simulink model "nncACCsystem_5_50"  (R2021a)
(part 13 of 14)

  "IW{5,4}(50,:)'" : Constant  Value=[0.1141432004020616342021554601160460151731967926025390625;-0.017584047457666528158082286381613812409341335296630859375;0.66805155463235965651591641289996914565563201904296875;-0.6136001546513243365410517071723006665706634521484375;0.95937034133340282071600313429371453821659088134765625;0.075971577456444838727378510156995616853237152099609375;0.5297921278961776891947010881267488002777099609375;0.12067691519441682557189920999007881619036197662353515625;-0.191581829978980433537572025670669972896575927734375;-0.1087005623838290524485472587912227027118206024169921875;0.0784168938973104356904286760254763066768646240234375;0.6065395454377213724228568025864660739898681640625;-0.346902780311276026647959724868997000157833099365234375;0.217804850814769912492607772946939803659915924072265625;-0.990997053395485050231172863277606666088104248046875;0.0857487248848738670137237249946338124573230743408203125;-0.05128831403013651979438947137168725021183490753173828125;-0.9629031136673800173042536698631010949611663818359375;-0.829893972023025838780085905455052852630615234375;-0.74057440662256468488777727543492801487445831298828125;0.5856000846022102468424463950213976204395294189453125;0.515406069917983433725794384372420608997344970703125;0.8084890601401026888339629294932819902896881103515625;0.21723000990280361133244468874181620776653289794921875;-0.211007213040456775843267678283154964447021484375;-0.52450505825967430606482366783893667161464691162109375;-0.7760978893070304973633710687863640487194061279296875;-0.2729152713620124348636863942374475300312042236328125;-0.7843894258724890544698382655042223632335662841796875;0.7267607104040860743765506413183175027370452880859375;0.06688400233054224430784273636163561604917049407958984375;-0.22242900136235022046093945391476154327392578125;-0.433234064722516354351000700262375175952911376953125;0.268465430229838819542464989353902637958526611328125;0.83968421280373828352594500756822526454925537109375;-0.300231039082238027049243100918829441070556640625;-0.50942280050992094775352825308800674974918365478515625;-0.072633643631129007900426586274988949298858642578125;-0.0176651529053561962001595020410604774951934814453125;-0.1689808965722979505752476825364283286035060882568359375;-0.61101340370974821514238328745705075562000274658203125;-0.92770092769464718163163752251421101391315460205078125;-0.6814966471176699958078870622557587921619415283203125;0.74963349363538289704678163616335950791835784912109375;0.471918139959748739187261890037916600704193115234375;0.42976609261675891016096784369437955319881439208984375;-0.2913539067186416975374640969675965607166290283203125;-0.26473179229769050468945579268620349466800689697265625;-0.1494398826271263747145212619216181337833404541015625;-0.0047963111412494228991132416695108986459672451019287109375]
      mask Display: e = 0.06;c1 = [120 150 230]/255;c2 = ([120 150 230]+0)/383;c3 = ([120 150 230]+128)/383;patch([0 1 1 0],[0 0 1 1],c1);patch([0 1 1 1-e 1-e 0+e],[0 0 1 1-e 0+e 0+e],c2);patch([0 0 1 1-e 0+e 0+e],[0 1 1 1-e 1-e 0+e],c3);plot([0 1 1 0 0],[0 0 1 1 0]);disp('weights');
  "IW{5,4}(6,:)'" : Constant  Value=[0.3562295317008794537372295962995849549770355224609375;-0.9594267744298006217462670974782668054103851318359375;-0.8561211729585240792772538043209351599216461181640625;-0.6858649005114350050149596427218057215213775634765625;0.693357420721138151264995030942372977733612060546875;0.6491811538530491976217717819963581860065460205078125;0.4650031948144783822129966210923157632350921630859375;-0.4006238615764019517229144184966571629047393798828125;-0.8360217807908802978289486418361775577068328857421875;-0.0467611414599111707701695195282809436321258544921875;-0.901853552230166055636573219089768826961517333984375;-0.350978204962510975661871270858682692050933837890625;-0.2877242832576334397032269407645799219608306884765625;0.0514980364986763472501252181245945394039154052734375;0.26081748415533212437367183156311511993408203125;0.3529120801958651743035488834721036255359649658203125;0.6029519225999704357121800057939253747463226318359375;-0.0818034610827227393059501991956494748592376708984375;0.134101733301195569225683357217349112033843994140625;-0.6303215523613399096092280160519294440746307373046875;-0.79676277486145608008882845751941204071044921875;0.4374804970924806024612507826532237231731414794921875;0.1479652196327256863384036478237248957157135009765625;0.0855815758666143011623717029578983783721923828125;-0.8378126628961728439293210612959228456020355224609375;-0.6633050510598119675620409907423891127109527587890625;-0.8438418931206477235917873258586041629314422607421875;-0.828178424658374989775211361120454967021942138671875;0.7593314799986021768063437775708734989166259765625;0.1850531885661881315030541372834704816341400146484375;0.01103491414841784035161253996193408966064453125;0.0433833817025632839659010642208158969879150390625;-0.3893360678296999832781466466258279979228973388671875;0.1383580395647197036623765598051249980926513671875;-0.2893368068265278481021596235223114490509033203125;0.6991119862498920145554848204483278095722198486328125;-0.8131628013724869763478864115313626825809478759765625;0.786580773429571333821286316378973424434661865234375;0.0515801109804245871970351799973286688327789306640625;-0.2752704126105511850397533635259605944156646728515625;-0.0373661458551948211237458963296376168727874755859375;0.4458566657836804392189833379234187304973602294921875;-0.656736574649199322806225609383545815944671630859375;0.2401126867635745565365823495085351169109344482421875;-0.8042628758426690893656996195204555988311767578125;-0.95927744782383772559342105523683130741119384765625;-0.82736867483109488574655188131146132946014404296875;-0.66927779776266316247301801922731101512908935546875;-0.0234373844901714090127597955870442092418670654296875;-0.0099647596443699359980428198468871414661407470703125]
      mask Display: e = 0.06;c1 = [120 150 230]/255;c2 = ([120 150 230]+0)/383;c3 = ([120 150 230]+128)/383;patch([0 1 1 0],[0 0 1 1],c1);patch([0 1 1 1-e 1-e 0+e],[0 0 1 1-e 0+e 0+e],c2);patch([0 0 1 1-e 0+e 0+e],[0 1 1 1-e 1-e 0+e],c3);plot([0 1 1 0 0],[0 0 1 1 0]);disp('weights');
  "IW{5,4}(7,:)'" : Constant  Value=[-0.501231035064013230595492132124491035938262939453125;-0.357691629081013429125590619150898419320583343505859375;-0.7900913539664988771704656755900941789150238037109375;0.2096838828164602208659061943762935698032379150390625;0.62382138299157607885803145109093748033046722412109375;0.1366901035758718296886371490472811274230480194091796875;-0.233367237568067320552245291764847934246063232421875;0.252547828187033640556791169728967361152172088623046875;0.7087636839718935988230441580526530742645263671875;-0.90527397696553568717803273102617822587490081787109375;0.6014760521333943898980578524060547351837158203125;-0.530859910497331721757063860422931611537933349609375;-0.38246638282558509391861889525898732244968414306640625;0.31591269256083831518111537661752663552761077880859375;-0.62210156570651020668805131208500824868679046630859375;-0.480663856403305889131161166005767881870269775390625;0.0945553776214251018306100604604580439627170562744140625;-0.1882986261857273191377970533721963874995708465576171875;0.152877254705158893699490363360382616519927978515625;-0.0699828261606157686625095948329544626176357269287109375;-0.58808697276489441119196044382988475263118743896484375;0.357367299668190085970564950912375934422016143798828125;0.70759581042943209272522153696627356112003326416015625;-0.042104488211461947588798437891455250792205333709716796875;-0.5940109083731683892182218187372200191020965576171875;0.85650981721000807311838798341341316699981689453125;0.3521252772321890045503778310376219451427459716796875;0.81358484949936660246549990915809758007526397705078125;-0.718740687327045879584375143167562782764434814453125;-0.331609948990100489307764064506045542657375335693359375;0.5977500263709998318262250904808752238750457763671875;-0.375894633733153238352997504989616572856903076171875;-0.80113567733840085338670178316533565521240234375;0.7216532547682579235015509766526520252227783203125;0.8335636424205983274760001222603023052215576171875;-0.4197666285151575582546001896844245493412017822265625;0.63216733030109562019305258218082599341869354248046875;-0.1751530510027360654223826941233710385859012603759765625;0.5914122117394067235096599688404239714145660400390625;0.1766025750526220294833734669737168587744235992431640625;0.353507921430033345000509825695189647376537322998046875;-0.884736247267077668965384873445145785808563232421875;0.0273307323542046898268154109246097505092620849609375;0.16360477382383231681473034768714569509029388427734375;-0.854591073876117324203960379236377775669097900390625;-0.55889232599558991143595676476252265274524688720703125;-0.850124795777536856888900729245506227016448974609375;0.9188706920610811845762100347201339900493621826171875;-0.0448718826156000449856264822301454842090606689453125;-0.071636817070096336923512581051909364759922027587890625]
      mask Display: e = 0.06;c1 = [120 150 230]/255;c2 = ([120 150 230]+0)/383;c3 = ([120 150 230]+128)/383;patch([0 1 1 0],[0 0 1 1],c1);patch([0 1 1 1-e 1-e 0+e],[0 0 1 1-e 0+e 0+e],c2);patch([0 0 1 1-e 0+e 0+e],[0 1 1 1-e 1-e 0+e],c3);plot([0 1 1 0 0],[0 0 1 1 0]);disp('weights');
  "IW{5,4}(8,:)'" : Constant  Value=[-0.835397376692058823977049542008899152278900146484375;-0.1863177926218158031446137101738713681697845458984375;0.947840470946463842238927099970169365406036376953125;-0.40320951499648050031510138069279491901397705078125;0.8429824173771149897760324165574274957180023193359375;0.189470039698699910246659783297218382358551025390625;-0.168120473083930743740666002850048243999481201171875;0.3850826533089504177809203611104749143123626708984375;-0.0568519217815877109245548126637004315853118896484375;0.8730703813938365254188056496786884963512420654296875;-0.76807973930514084059950619121082127094268798828125;0.985893388329737607733704862766899168491363525390625;0.957910694214652469469228890375234186649322509765625;0.567445330118751645187558096949942409992218017578125;-0.073250503132566091579747080686502158641815185546875;-0.2572748304222669535334944157511927187442779541015625;-0.9233194436739300403615970935788936913013458251953125;0.693241279306989088837553936173208057880401611328125;-0.7155330006054583247276923430035822093486785888671875;-0.6614285298641149335452382729272358119487762451171875;-0.1588593543599252644327179950778372585773468017578125;0.2010344578168161699949223475414328277111053466796875;-0.1237958922126274341479756913031451404094696044921875;-0.1151649177598332851601981019484810531139373779296875;-0.49354322715469667315346669056452810764312744140625;-0.702844637054997445346771201002411544322967529296875;0.65052194756236314532316100667230784893035888671875;-0.333695281534292842451350225019268691539764404296875;0.761133946108828229881737570394761860370635986328125;-0.1631563584736659411333903335616923868656158447265625;-0.75700179216406393578608913230709731578826904296875;-0.449358337881843095118483688565902411937713623046875;-0.790585520472188107987676630727946758270263671875;-0.5439977754440203927543961981427855789661407470703125;-0.4510031405965089223997210865491069853305816650390625;-0.4421511393272237189222551023703999817371368408203125;-0.025489463464555495164631793159060180187225341796875;-0.3536782445976800470788248276221565902233123779296875;-0.307989351103557407185462579946033656597137451171875;-0.5623830419630575505607339437119662761688232421875;0.58988972588036858724080957472324371337890625;-0.4032539307774827275210327570675872266292572021484375;0.4908366314473247005167877432540990412235260009765625;0.003280045227161298981854997691698372364044189453125;-0.3422400378460412895265108090825378894805908203125;-0.721939022319336487498731003142893314361572265625;-0.1268024164893539751375328705762512981891632080078125;-0.5045654316656384974493221307056955993175506591796875;-0.9188881947066196431705975555814802646636962890625;0.2464410919689814516431169977295212447643280029296875]
      mask Display: e = 0.06;c1 = [120 150 230]/255;c2 = ([120 150 230]+0)/383;c3 = ([120 150 230]+128)/383;patch([0 1 1 0],[0 0 1 1],c1);patch([0 1 1 1-e 1-e 0+e],[0 0 1 1-e 0+e 0+e],c2);patch([0 0 1 1-e 0+e 0+e],[0 1 1 1-e 1-e 0+e],c3);plot([0 1 1 0 0],[0 0 1 1 0]);disp('weights');
  "IW{5,4}(9,:)'" : Constant  Value=[0.125263869427104879150647320784628391265869140625;-0.26892420971510777594204455454018898308277130126953125;-0.336354899111460048377608700320706702768802642822265625;-0.904315649536205246050712958094663918018341064453125;-0.88276543462096912495695733014144934713840484619140625;0.1946548813334317562517838950952864252030849456787109375;-0.507868156492297107007516387966461479663848876953125;0.9092107987620712261644939644611440598964691162109375;0.721076330649817354156994042568840086460113525390625;0.6995281039499550157501062130904756486415863037109375;0.768981913009282092019702758989296853542327880859375;0.8510055912506089281777121868799440562725067138671875;0.9110055475525749013598897363408468663692474365234375;-0.1512888880825329074308882582045043818652629852294921875;0.9864111784332727506097171499277465045452117919921875;0.45705781453436333805484537151642143726348876953125;0.0582522255673158240174558386570424772799015045166015625;-0.2783090350975634397201474712346680462360382080078125;-0.2050213130668951944102218476473353803157806396484375;0.9062783858765453004480150411836802959442138671875;-0.2275372272443366428174016391494660638272762298583984375;-0.74975055782701927054034740649512968957424163818359375;-0.00167456629070278297140295098444084942457266151905059814453125;-0.68684648197941322589343826621188782155513763427734375;0.274321371547895154208163148723542690277099609375;-0.8326166588818690872386696355533786118030548095703125;0.3492783513319797084051288038608618080615997314453125;-0.352424262757165263071357230728608556091785430908203125;-0.56161177963944464153200897271744906902313232421875;0.60711015775531829152811269523226656019687652587890625;0.653327372178704735006249393336474895477294921875;-0.2734280753837075028656045105890370905399322509765625;0.9471567103199796111567820844356901943683624267578125;0.0691495345151629248192648447002284228801727294921875;-0.55269637080893829761407687328755855560302734375;0.8364099330009135968566624796949326992034912109375;0.93565814778570077780983638149336911737918853759765625;0.7440300375040942437721014357521198689937591552734375;-0.6031580020371298811454607857740484178066253662109375;0.54771961519984102562119687718222849071025848388671875;0.356311952272694298926580813713371753692626953125;-0.23858451746665476633779690018855035305023193359375;0.369998883276509094031325730611570179462432861328125;-0.9154668776852885603290133076370693743228912353515625;0.32110909552635202857118201791308820247650146484375;0.397166094851536310983419753029011189937591552734375;0.097140944587528199605230838642455637454986572265625;-0.251072166322450052167170042594079859554767608642578125;-0.8427613145815346928912958901491947472095489501953125;-0.155964300466448435589228438402642495930194854736328125]
      mask Display: e = 0.06;c1 = [120 150 230]/255;c2 = ([120 150 230]+0)/383;c3 = ([120 150 230]+128)/383;patch([0 1 1 0],[0 0 1 1],c1);patch([0 1 1 1-e 1-e 0+e],[0 0 1 1-e 0+e 0+e],c2);patch([0 0 1 1-e 0+e 0+e],[0 1 1 1-e 1-e 0+e],c3);plot([0 1 1 0 0],[0 0 1 1 0]);disp('weights');
  Mux : Mux  Inputs=50
      mask Display: e = 0.06;c1 = [120 150 230]/255;c2 = ([120 150 230]+0)/383;c3 = ([120 150 230]+128)/383;patch([0 1 1 0],[0 0 1 1],c1);patch([0 1 1 1-e 1-e 0+e],[0 0 1 1-e 0+e 0+e],c2);patch([0 0 1 1-e 0+e 0+e],[0 1 1 1-e 1-e 0+e],c3);plot([0 1 1 0 0],[0 0 1 1 0]);disp('Mux');
  dotprod{1..50} (50 alike) : neural/Weight Functions/dotprod
  "lz{5,4}" : Outport
      mask Display: e = 0.06;c1 = [120 230 180]/255;c2 = ([120 230 180]+0)/(256+128);c3 = ([120 230 180]+128)/(256+128);patch([0 1 1 0],[0 0 1 1],c1);patch([0 1 1 1-e 1-e 0+e],[0 0 1 1-e 0+e 0+e],c2);patch([0 0 1 1-e 0+e 0+e],[0 1 1 1-e 1-e 0+e],c3);plot([0 1 1 0 0],[0 0 1 1 0]);
  wires:
  Mux/1 -> "lz{5,4}"/1
  dotprod50/1 -> Mux/50
  "IW{5,4}(50,:)'"/1 -> dotprod50/1
  dotprod49/1 -> Mux/49
  "IW{5,4}(49,:)'"/1 -> dotprod49/1
  dotprod48/1 -> Mux/48
  "IW{5,4}(48,:)'"/1 -> dotprod48/1
  dotprod47/1 -> Mux/47
  "IW{5,4}(47,:)'"/1 -> dotprod47/1
  dotprod46/1 -> Mux/46
  "IW{5,4}(46,:)'"/1 -> dotprod46/1
  dotprod45/1 -> Mux/45
  "IW{5,4}(45,:)'"/1 -> dotprod45/1
  dotprod44/1 -> Mux/44
  "IW{5,4}(44,:)'"/1 -> dotprod44/1
  dotprod43/1 -> Mux/43
  "IW{5,4}(43,:)'"/1 -> dotprod43/1
  dotprod42/1 -> Mux/42
  "IW{5,4}(42,:)'"/1 -> dotprod42/1
  dotprod41/1 -> Mux/41
  "IW{5,4}(41,:)'"/1 -> dotprod41/1
  dotprod40/1 -> Mux/40
  "IW{5,4}(40,:)'"/1 -> dotprod40/1
  dotprod39/1 -> Mux/39
  "IW{5,4}(39,:)'"/1 -> dotprod39/1
  dotprod38/1 -> Mux/38
  "IW{5,4}(38,:)'"/1 -> dotprod38/1
  dotprod37/1 -> Mux/37
  "IW{5,4}(37,:)'"/1 -> dotprod37/1
  dotprod36/1 -> Mux/36
  "IW{5,4}(36,:)'"/1 -> dotprod36/1
  dotprod35/1 -> Mux/35
  "IW{5,4}(35,:)'"/1 -> dotprod35/1
  dotprod34/1 -> Mux/34
  "IW{5,4}(34,:)'"/1 -> dotprod34/1
  dotprod33/1 -> Mux/33
  "IW{5,4}(33,:)'"/1 -> dotprod33/1
  dotprod32/1 -> Mux/32
  "IW{5,4}(32,:)'"/1 -> dotprod32/1
  dotprod31/1 -> Mux/31
  "IW{5,4}(31,:)'"/1 -> dotprod31/1
  dotprod30/1 -> Mux/30
  "IW{5,4}(30,:)'"/1 -> dotprod30/1
  dotprod29/1 -> Mux/29
  "IW{5,4}(29,:)'"/1 -> dotprod29/1
  dotprod28/1 -> Mux/28
  "IW{5,4}(28,:)'"/1 -> dotprod28/1
  dotprod27/1 -> Mux/27
  "IW{5,4}(27,:)'"/1 -> dotprod27/1
  dotprod26/1 -> Mux/26
  "IW{5,4}(26,:)'"/1 -> dotprod26/1
  dotprod25/1 -> Mux/25
  "IW{5,4}(25,:)'"/1 -> dotprod25/1
  dotprod24/1 -> Mux/24
  "IW{5,4}(24,:)'"/1 -> dotprod24/1
  dotprod23/1 -> Mux/23
  "IW{5,4}(23,:)'"/1 -> dotprod23/1
  dotprod22/1 -> Mux/22
  "IW{5,4}(22,:)'"/1 -> dotprod22/1
  dotprod21/1 -> Mux/21
  "IW{5,4}(21,:)'"/1 -> dotprod21/1
  dotprod20/1 -> Mux/20
  "IW{5,4}(20,:)'"/1 -> dotprod20/1
  dotprod19/1 -> Mux/19
  "IW{5,4}(19,:)'"/1 -> dotprod19/1
  dotprod18/1 -> Mux/18
  "IW{5,4}(18,:)'"/1 -> dotprod18/1
  dotprod17/1 -> Mux/17
  "IW{5,4}(17,:)'"/1 -> dotprod17/1
  dotprod16/1 -> Mux/16
  "IW{5,4}(16,:)'"/1 -> dotprod16/1
  dotprod15/1 -> Mux/15
  "IW{5,4}(15,:)'"/1 -> dotprod15/1
  dotprod14/1 -> Mux/14
  "IW{5,4}(14,:)'"/1 -> dotprod14/1
  dotprod13/1 -> Mux/13
  "IW{5,4}(13,:)'"/1 -> dotprod13/1
  dotprod12/1 -> Mux/12
  "IW{5,4}(12,:)'"/1 -> dotprod12/1
  dotprod11/1 -> Mux/11
  "IW{5,4}(11,:)'"/1 -> dotprod11/1
  dotprod10/1 -> Mux/10
  "IW{5,4}(10,:)'"/1 -> dotprod10/1
  dotprod9/1 -> Mux/9
  "IW{5,4}(9,:)'"/1 -> dotprod9/1
  dotprod8/1 -> Mux/8
  "IW{5,4}(8,:)'"/1 -> dotprod8/1
  dotprod7/1 -> Mux/7
  "IW{5,4}(7,:)'"/1 -> dotprod7/1
  dotprod6/1 -> Mux/6
  "IW{5,4}(6,:)'"/1 -> dotprod6/1
  dotprod5/1 -> Mux/5
  "IW{5,4}(5,:)'"/1 -> dotprod5/1
  dotprod4/1 -> Mux/4
  "IW{5,4}(4,:)'"/1 -> dotprod4/1
  dotprod3/1 -> Mux/3
  "IW{5,4}(3,:)'"/1 -> dotprod3/1
  dotprod2/1 -> Mux/2
  "IW{5,4}(2,:)'"/1 -> dotprod2/1
  dotprod1/1 -> Mux/1
  "ad{5,4}"/1 -> dotprod50/2, dotprod49/2, dotprod48/2, dotprod47/2, dotprod46/2, dotprod45/2, dotprod44/2, dotprod43/2, dotprod42/2, dotprod41/2, dotprod40/2, dotprod39/2, dotprod38/2, dotprod37/2, dotprod36/2, dotprod35/2, dotprod34/2, dotprod33/2, dotprod32/2, dotprod31/2, dotprod30/2, dotprod29/2, dotprod28/2, dotprod27/2, dotprod26/2, dotprod25/2, dotprod24/2, dotprod23/2, dotprod22/2, dotprod21/2, dotprod20/2, dotprod19/2, dotprod18/2, dotprod17/2, dotprod16/2, dotprod15/2, dotprod14/2, dotprod13/2, dotprod12/2, dotprod11/2, dotprod10/2, dotprod9/2, dotprod8/2, dotprod7/2, dotprod6/2, dotprod5/2, dotprod4/2, dotprod3/2, dotprod2/2, dotprod1/2
  "IW{5,4}(1,:)'"/1 -> dotprod1/1
